simulink library "NOODL_translational_PTO_v2"  (R2024a)
settings: Solver=VariableStepAuto  StartTime=0.0  StopTime=10.0  RelTol=1e-3
undefined symbols (not defined in the file): pto
libraries: WECSim_Lib_PTOs x1, hose_pump_unit_v3 x1
settings Model: Creator=cmmcguir  LastModifiedBy=Carson

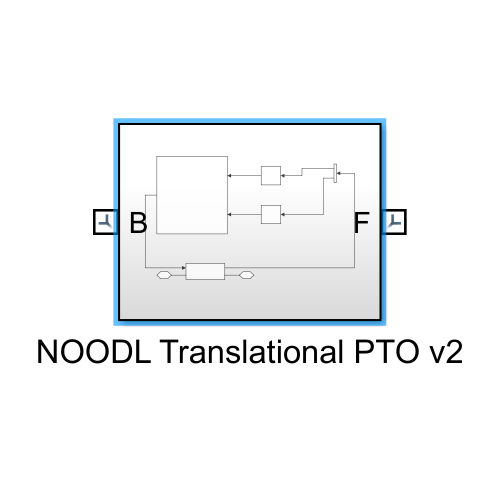
[thumbnail: Simulink's stored preview of the top-level diagram]
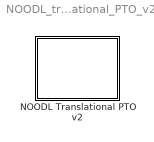
== system NOODL_translational_PTO_v2 ==
  NOODL Translational PTO v2 : Subsystem

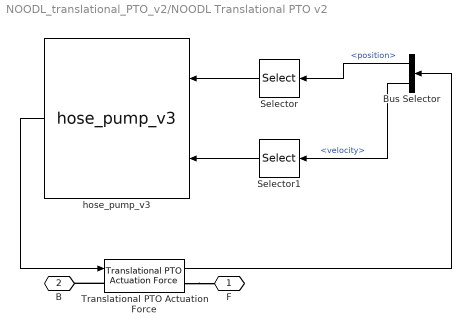
== system NOODL_translational_PTO_v2/NOODL Translational PTO v2 ==
  Bus Selector : BusSelector  OutputSignals=position,velocity
  Selector : Selector  InputPortWidth=6  IndexOptions=Index vector (dialog)  Indices=[3]  OutputSizes=1
  Selector1 : Selector  InputPortWidth=6  IndexOptions=Index vector (dialog)  Indices=[3]  OutputSizes=1
  Translational PTO Actuation Force : WECSim_Lib_PTOs/Translational PTO Actuation Force  pto=pto(1)  loc="0  0  0"  stiffness=0  damping=0  equilibriumPosition=0  pretension=0  displacement=0 0 0  y=0 1 0  z=0 0 1  upperLimitSpecify=off  upperLimitBound=0  upperLimitTransitionRegionWidth=0  upperLimitStiffness=0  upperLimitDamping=0  lowerLimitSpecify=off  lowerLimitBound=0  lowerLimitTransitionRegionWidth=0  lowerLimitStiffness=0  lowerLimitDamping=0
      settings: AttributesFormatString=%<pto>
  hose_pump_v3 : hose_pump_unit_v3/hose_pump_v3  SystemSampleTime=-1  VariantActivationTime=update diagram  AllowFlexibleInterface=on  Latency=0  AutoFrameSizeCalculation=off
  F : PMIOPort  Side=Right
  B : PMIOPort  Port=2  Side=Left
  wires:
  Translational PTO Actuation Force/1 -> Bus Selector/1
  hose_pump_v3/1 -> Translational PTO Actuation Force/1
  Bus Selector/1 -> Selector/1  "<position>"
  Bus Selector/2 -> Selector1/1  "<velocity>"
  Selector/1 -> hose_pump_v3/1
  Selector1/1 -> hose_pump_v3/2
  connections:
  Translational PTO Actuation Force/RConn1 -- F/RConn1
  Translational PTO Actuation Force/LConn1 -- B/RConn1
